simulink model "robot_model"  (R2025a)
settings: Solver=FixedStepDiscrete  StartTime=0.0  StopTime=inf  FixedStep=0.01  RelTol=1e-3  EnableMultiTasking=on
PreLoadFcn:
  | frs = FrankaRobotSettings;
undefined symbols (not defined in the file): Effector, End
libraries: franka_simulink x5
settings Model: SimulationMode=external  ExtModeTrigDuration=10000  Creator=vasi_ko  LastModifiedBy=kvasios
settings SolverCC: ConcurrentTasks=on  AlgebraicLoopSolver=TrustRegion  AutoInsertRateTranBlk=on
settings DataIOCC: LimitDataPoints=on  SaveFormat=Array  ReturnWorkspaceOutputs=off
settings OptimizationCC: EnhancedBackFolding=on  PassReuseOutputArgsAs=Individual arguments  ZeroExternalMemoryAtStartup=off  ZeroInternalMemoryAtStartup=off  MaxStackSize=200000  OptimizeBlockOrder=speed  DifferentSizesBufferReuse=on  OptimizationCustomize=off  EfficientTunableParamExpr=on
settings DebuggingCC: SolverPrmCheckMsg=warning  ParameterTunabilityLossMsg=error  UnconnectedInputMsg=warning  UnconnectedOutputMsg=warning  UnconnectedLineMsg=warning  SFUnexpectedBacktrackingDiag=warning  SFNoUnconditionalDefaultTransitionDiag=warning  SFExecutionAtInitializationDiag=none  ArithmeticOperatorsInVariantConditions=warning
settings HardwareCC: ProdBitPerLong=64.0  ProdLargestAtomicInteger=LongLong  ProdLargestAtomicFloat=Double  ProdLongLongMode=on  ProdHWDeviceType=ARM Compatible->ARM Cortex-A (64-bit)
settings ModelReferenceCC: EnableRefExpFcnMdlSchedulingChecks=on  PropagateSignalLabelsOutOfModel=off
settings SFSimCC: SimUseLocalCustomCode=off  MATLABDynamicMemAlloc=off  CustomCodeUndefinedFunction=UseInterfaceOnly  SimTargetLang=C++  SimDLTargetLibrary=mkl-dnn
settings RTWCC: SystemTargetFile=ert.tlc  HardwareBoard=NVIDIA Jetson  TLCOptions="-aInlineSetEventsForThisBaseRateFcn=TLC_FALSE -aSuppressMultiTaskScheduler=TLC_FALSE  -aRateBasedStepFcn=0"  TemplateMakefile=ert_default_tmf  RTWVerbose=off  RTWUseLocalCustomCode=off  BuildConfiguration=Faster Runs  TargetLang=C++  GPUComputeCapability=3.5  DLArmComputeVersion=19.05  Description=Embedded Coder
settings CodeAppCC: ForceParamTrailComments=on  IgnoreCustomStorageClasses=off  OperatorAnnotations=on  SimulinkDataObjDesc=on  SFDataObjDesc=on  InsertBlockDesc=on
settings ERTTargetCC: ExtModeTransport=2.0  InlinedParameterPlacement=Hierarchical  RootIOFormat=Structure reference  TargetLangStandard=C++14 (ISO)
settings ConfigComp: CovMetricSettings=dw  CovSaveCumulativeToWorkspaceVar=on  CovSaveSingleToWorkspaceVar=on  CovExternalEMLEnable=off  CovSFcnEnable=off

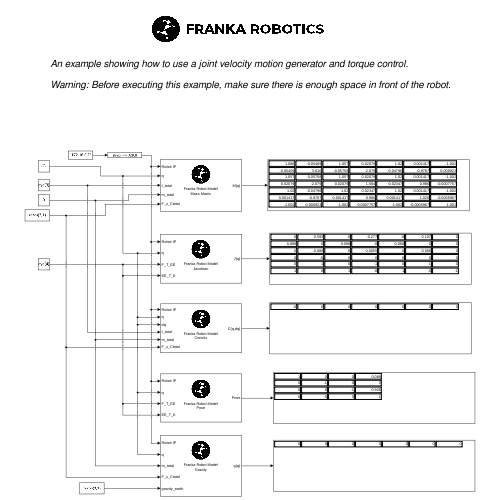
[thumbnail: Simulink's stored preview of the top-level diagram]
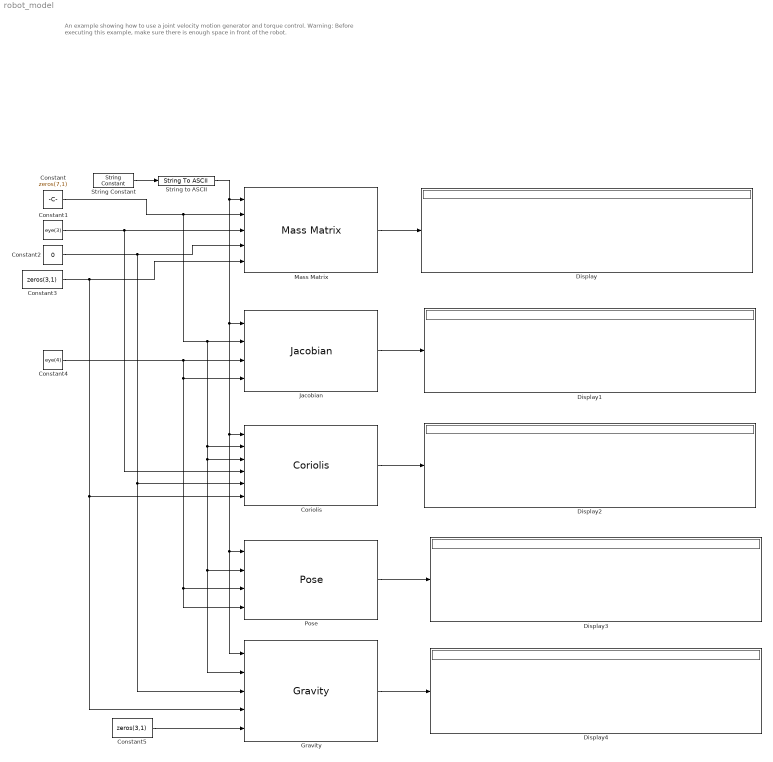
== system robot_model ==
  note: An example showing how to use a joint velocity motion generator and torque control.
      |
      | Warning: Before executing this example, make sure there is enough space in front of the robot.
  Constant : Constant  Value=zeros(7,1)
  Constant1 : Constant  Value=eye(3)
  Constant2 : Constant  Value=0
  Constant3 : Constant  Value=zeros(3,1)
  Constant4 : Constant  Value=eye(4)
  Constant5 : Constant  Value=zeros(3,1)
  Coriolis : franka_simulink/Robot Model/Coriolis
      settings: SourceProductName=Franka Robotics Simulink Support Package
  Display{,1..4} (5 alike) : Display
  Gravity : franka_simulink/Robot Model/Gravity  earth_gravity=on
      settings: SourceProductName=Franka Robotics Simulink Support Package
  Jacobian : franka_simulink/Robot Model/Jacobian  jacobian_type=Zero Jacobian  frame=End-Effector
      settings: SourceProductName=Franka Robotics Simulink Support Package
  Mass Matrix : franka_simulink/Robot Model/Mass Matrix
      settings: SourceProductName=Franka Robotics Simulink Support Package
  Pose : franka_simulink/Robot Model/Pose  frame=End-Effector
      settings: SourceProductName=Franka Robotics Simulink Support Package
  String Constant : StringConstant  String="\"172.16.0.2\""
  String to ASCII : StringToASCII  OutputVectorSize=16
  wires:
  Mass Matrix/1 -> Display/1
  String to ASCII/1 -> Pose/1, Gravity/1, Coriolis/1, Jacobian/1, Mass Matrix/1
  String Constant/1 -> String to ASCII/1
  Constant/1 -> Coriolis/3, Gravity/2, Pose/2, Coriolis/2, Jacobian/2, Mass Matrix/2
  Constant1/1 -> Coriolis/4, Mass Matrix/3
  Constant2/1 -> Gravity/3, Coriolis/5, Mass Matrix/4
  Constant3/1 -> Gravity/4, Coriolis/6, Mass Matrix/5
  Jacobian/1 -> Display1/1
  Constant4/1 -> Jacobian/3, Pose/4, Pose/3, Jacobian/4
  Coriolis/1 -> Display2/1
  Pose/1 -> Display3/1
  Gravity/1 -> Display4/1
  Constant5/1 -> Gravity/5
